simulink subsystem "NoElectrical"  (R2023a)
settings: Solver=VariableStepAuto  StartTime=0.0  StopTime=10.0  RelTol=1e-3
settings Model: Creator=The MathWorks, Inc.  LastModifiedBy=The MathWorks, Inc.

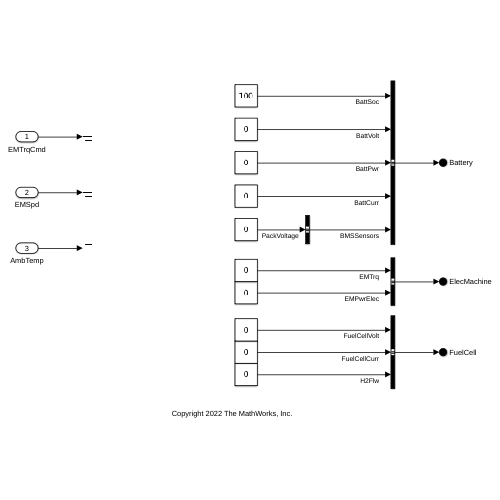
[thumbnail: Simulink's stored preview of the top-level diagram]
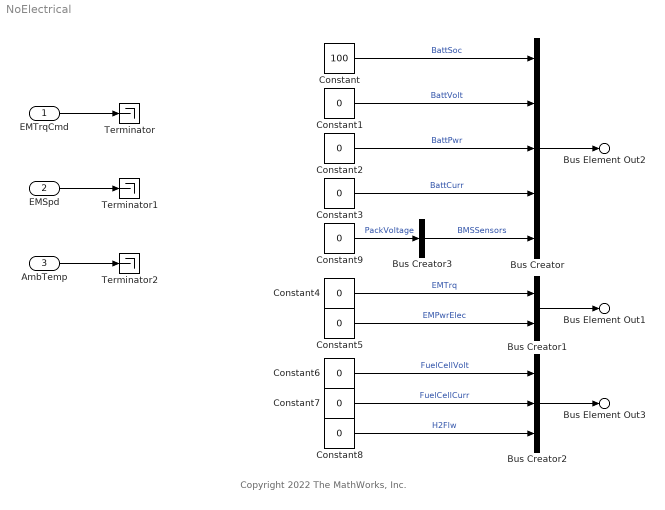
== system NoElectrical ==
  note: Copyright 2022 The MathWorks, Inc.
  EMTrqCmd : Inport
  EMSpd : Inport  Port=2
  AmbTemp : Inport  Port=3
  Bus Creator : BusCreator  Inputs=5
  Bus Creator1 : BusCreator  Inputs=2
  Bus Creator2 : BusCreator  Inputs=3
  Bus Creator3 : BusCreator  Inputs=1
  Constant : Constant  Value=100  SampleTime=-1
  Constant{1..9} (9 alike) : Constant  Value=0  SampleTime=-1
  Terminator : Terminator
  Terminator1 : Terminator
  Terminator2 : Terminator
  Bus Element Out2 : Outport  PortName=Battery
  Bus Element Out1 : Outport  Port=2  PortName=ElecMachine
  Bus Element Out3 : Outport  Port=3  PortName=FuelCell
  wires:
  Constant5/1 -> Bus Creator1/2  "EMPwrElec"
  Bus Creator2/1 -> Bus Element Out3/1
  Bus Creator1/1 -> Bus Element Out1/1
  Bus Creator/1 -> Bus Element Out2/1
  Constant1/1 -> Bus Creator/2  "BattVolt"
  Constant/1 -> Bus Creator/1  "BattSoc"
  Constant6/1 -> Bus Creator2/1  "FuelCellVolt"
  Constant7/1 -> Bus Creator2/2  "FuelCellCurr"
  Constant3/1 -> Bus Creator/4  "BattCurr"
  Constant4/1 -> Bus Creator1/1  "EMTrq"
  EMSpd/1 -> Terminator1/1
  AmbTemp/1 -> Terminator2/1
  Constant8/1 -> Bus Creator2/3  "H2Flw"
  EMTrqCmd/1 -> Terminator/1
  Constant2/1 -> Bus Creator/3  "BattPwr"
  Bus Creator3/1 -> Bus Creator/5  "BMSSensors"
  Constant9/1 -> Bus Creator3/1  "PackVoltage"
